simulink model "PF_implementacion_OnOff"  (R2023a)
settings: Solver=ode15s  StartTime=0.0  StopTime=t_sim  RelTol=1e-3
values from neighbouring files (symbols this model uses):
  F_in_fin = F_in    (= 2.9922)    [PF_CP_Completo_Level2.m]    (also in PF_CP_Completo_OnOff.m = 2.9843; PF_CP_Completo_OnOff_Flujo.m = 2.9843; PF_CP_Completo_OnOff_Full.m = 2.9843; PF_CP_Completo_OnOff_Intensidad.m = 2.9843)
  F_in_ini = F_in    (= 2.9922)    [PF_CP_Completo_Level2.m]    (also in PF_CP_Completo_OnOff.m = 2.9843; PF_CP_Completo_OnOff_Flujo.m = 2.9843; PF_CP_Completo_OnOff_Full.m = 2.9843; PF_CP_Completo_OnOff_Intensidad.m = 2.9843)
  I0_in_fin = I0_in    (= 200)    [PF_CP_Completo_Level2.m]    (also in PF_CP_Completo_OnOff.m; PF_CP_Completo_OnOff_Flujo.m; PF_CP_Completo_OnOff_Full.m; PF_CP_Completo_OnOff_Intensidad.m)
  I0_in_ini = I0_in    (= 200)    [PF_CP_Completo_Level2.m]    (also in PF_CP_Completo_OnOff.m; PF_CP_Completo_OnOff_Flujo.m; PF_CP_Completo_OnOff_Full.m; PF_CP_Completo_OnOff_Intensidad.m)
  L_in_fin = L_in    (= 0)    [PF_CP_Completo_Level2.m]    (also in PF_CP_Completo_OnOff.m; PF_CP_Completo_OnOff_Flujo.m; PF_CP_Completo_OnOff_Full.m; PF_CP_Completo_OnOff_Intensidad.m)
  L_in_ini = L_in    (= 0)    [PF_CP_Completo_Level2.m]    (also in PF_CP_Completo_OnOff.m; PF_CP_Completo_OnOff_Flujo.m; PF_CP_Completo_OnOff_Full.m; PF_CP_Completo_OnOff_Intensidad.m)
  Q_in_fin = Q_in    (= 0)    [PF_CP_Completo_Level2.m]    (also in PF_CP_Completo_OnOff.m; PF_CP_Completo_OnOff_Flujo.m; PF_CP_Completo_OnOff_Full.m; PF_CP_Completo_OnOff_Intensidad.m)
  Q_in_ini = Q_in    (= 0)    [PF_CP_Completo_Level2.m]    (also in PF_CP_Completo_OnOff.m; PF_CP_Completo_OnOff_Flujo.m; PF_CP_Completo_OnOff_Full.m; PF_CP_Completo_OnOff_Intensidad.m)
  S1_in_fin = S1_in*1.5    (= 90)    [PF_CP_Completo_Level2.m]    (also in PF_CP_Completo_OnOff.m = 66; PF_CP_Completo_OnOff_Flujo.m; PF_CP_Completo_OnOff_Full.m; PF_CP_Completo_OnOff_Intensidad.m = 60)
  S1_in_ini = S1_in    (= 60)    [PF_CP_Completo_Level2.m]    (also in PF_CP_Completo_OnOff.m; PF_CP_Completo_OnOff_Flujo.m; PF_CP_Completo_OnOff_Full.m; PF_CP_Completo_OnOff_Intensidad.m)
  S2_in_fin = S2_in    (= 20)    [PF_CP_Completo_Level2.m]    (also in PF_CP_Completo_OnOff.m; PF_CP_Completo_OnOff_Flujo.m; PF_CP_Completo_OnOff_Full.m; PF_CP_Completo_OnOff_Intensidad.m)
  S2_in_ini = S2_in    (= 20)    [PF_CP_Completo_Level2.m]    (also in PF_CP_Completo_OnOff.m; PF_CP_Completo_OnOff_Flujo.m; PF_CP_Completo_OnOff_Full.m; PF_CP_Completo_OnOff_Intensidad.m)
  t_step = 10000    [PF_CP_Completo_Level2.m]    (also in PF_CP_Completo_OnOff.m; PF_CP_Completo_OnOff_Flujo.m = 1000; PF_CP_Completo_OnOff_Full.m = 2000; PF_CP_Completo_OnOff_Intensidad.m = 1000)
  x_in_fin = x_in    (= 0)    [PF_CP_Completo_Level2.m]    (also in PF_CP_Completo_OnOff.m; PF_CP_Completo_OnOff_Flujo.m; PF_CP_Completo_OnOff_Full.m; PF_CP_Completo_OnOff_Intensidad.m)
  x_in_ini = x_in    (= 0)    [PF_CP_Completo_Level2.m]    (also in PF_CP_Completo_OnOff.m; PF_CP_Completo_OnOff_Flujo.m; PF_CP_Completo_OnOff_Full.m; PF_CP_Completo_OnOff_Intensidad.m)
settings Model: Creator=ja616  LastModifiedBy=ja616

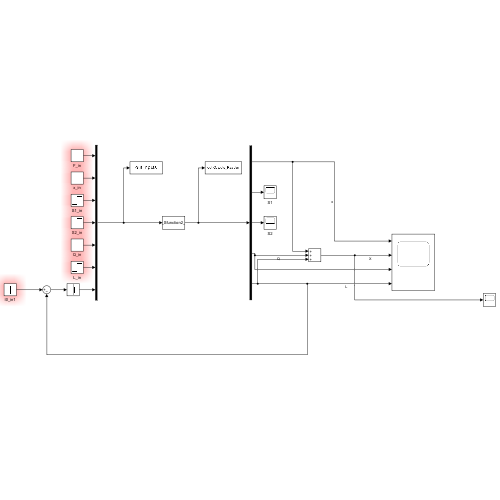
[thumbnail: Simulink's stored preview of the top-level diagram]
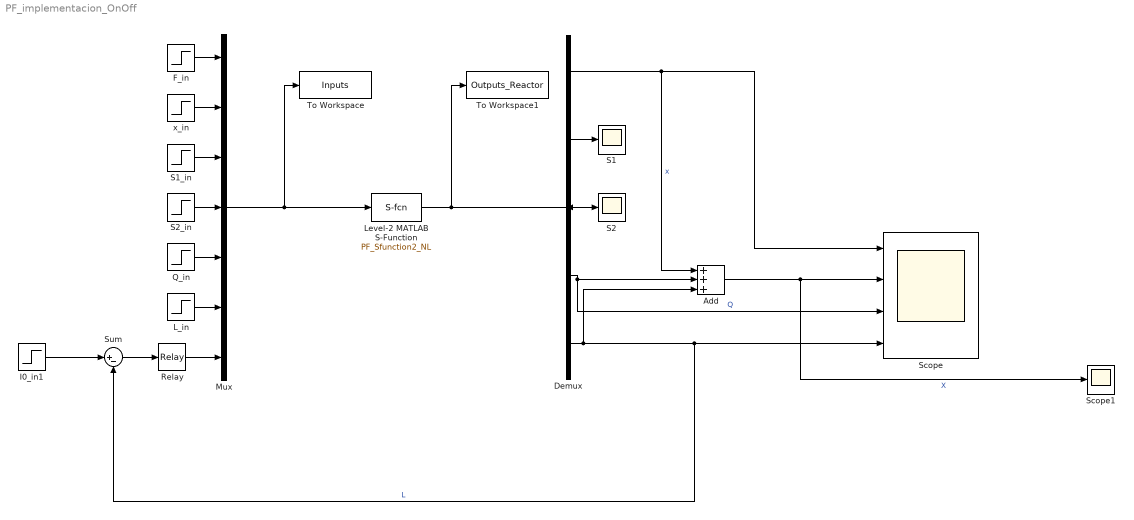
== system PF_implementacion_OnOff ==
  Add : Sum  Inputs=+++
  Demux : Demux  Outputs=5
  F_in : Step  Time=t_step  Before=F_in_ini  After=F_in_fin  SampleTime=0
  I0_in1 : Step  Time=t_step  Before=I0_in_ini  After=I0_in_fin  SampleTime=0
  L_in : Step  Time=t_step  Before=L_in_ini  After=L_in_fin  SampleTime=0
  Level-2 MATLAB S-Function : M-S-Function  FunctionName=PF_Sfunction2_NL
  Mux : Mux  Inputs=7
  Q_in : Step  Time=t_step  Before=Q_in_ini  After=Q_in_fin  SampleTime=0
  Relay : Relay
  S1 : Scope
  S1_in : Step  Time=t_step  Before=S1_in_ini  After=S1_in_fin  SampleTime=0
  S2 : Scope
  S2_in : Step  Time=t_step  Before=S2_in_ini  After=S2_in_fin  SampleTime=0
  Scope : Scope  NumInputPorts=4
  Scope1 : Scope
  Sum : Sum  Inputs=|+-
  To Workspace : ToWorkspace  VariableName=Inputs  SaveFormat=Timeseries  SampleTime=-1
  To Workspace1 : ToWorkspace  VariableName=Outputs_Reactor  SaveFormat=Timeseries  SampleTime=-1
  x_in : Step  Time=t_step  Before=x_in_ini  After=x_in_fin  SampleTime=0
  wires:
  F_in/1 -> Mux/1
  Mux/1 -> Level-2 MATLAB S-Function/1, To Workspace/1
  L_in/1 -> Mux/6
  S2_in/1 -> Mux/4
  S1_in/1 -> Mux/3
  Level-2 MATLAB S-Function/1 -> Demux/1, To Workspace1/1
  Q_in/1 -> Mux/5
  x_in/1 -> Mux/2
  Demux/1 -> Scope/1, Add/1  "x"
  Demux/2 -> S1/1
  Demux/3 -> S2/1
  Demux/4 -> Scope/3, Add/2  "Q"
  Demux/5 -> Add/3, Sum/2, Scope/4  "L"
  Add/1 -> Scope1/1, Scope/2  "X"
  I0_in1/1 -> Sum/1
  Sum/1 -> Relay/1
  Relay/1 -> Mux/7
